simulink model "Test_Position_Joints"  (Simulink 6.5)
settings: Solver=FixedStepDiscrete  StartTime=0.0  StopTime=inf  FixedStep=0.025  RelTol=1e-3
libraries: xpclib x8, simulink x4
settings Model: Creator=ilMaggia  LastModifiedBy=ilMaggia
settings DebuggingCC: MultiTaskDSMMsg=warning  MultiTaskCondExecSysMsg=none
settings RTWCC: SystemTargetFile=rtwin.tlc  TemplateMakefile=rtwin.tmf  Description=Real-Time Windows Target  ProcessScript=rtwin_make_rtw_hook  IncludeERTFirstTime=on
settings RTWinTargetCC: TargetFcnLib=ansi_tfl_tmw.mat  GenFloatMathFcnCalls=ANSI_C  ModelReferenceCompliant=off  CCOptimize=on

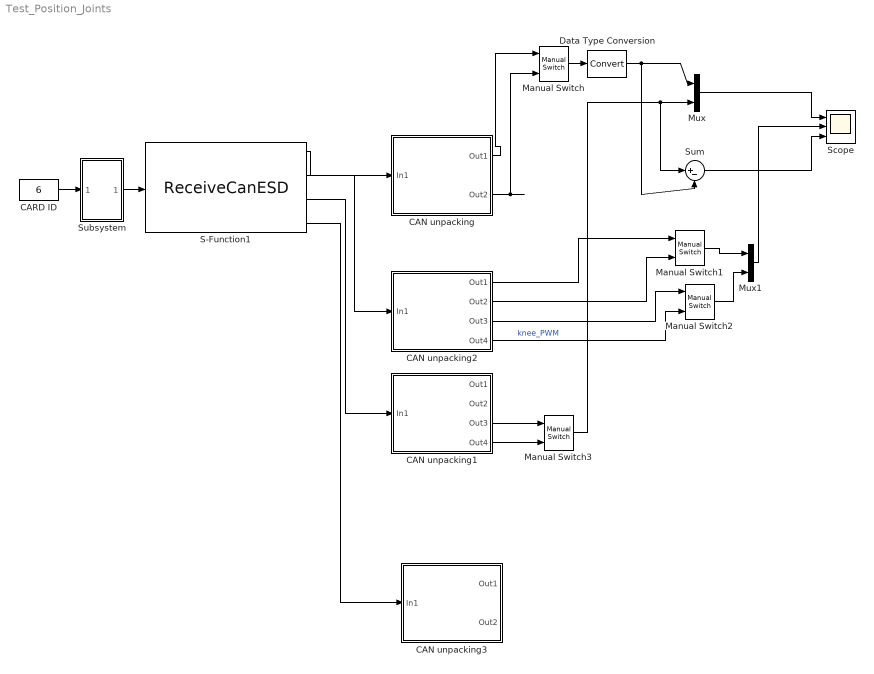
== system Test_Position_Joints ==
  CAN unpacking : Subsystem
  CAN unpacking1 : Subsystem
  CAN unpacking2 : Subsystem
  CAN unpacking3 : Subsystem
  CARD ID : Constant  Value=6  OutDataType=sfix(16)  ConRadixGroup=Use specified scaling  OutScaling=2^0  SampleTime=inf  FramePeriod=inf
  Data Type Conversion : DataTypeConversion
  Manual Switch{,1..3} (4 alike) : simulink/Signal Routing/Manual Switch  SystemSampleTime=-1  sw=1  action=0
  Mux : Mux  Inputs=2
  Mux1 : Mux  Inputs=2
  S-Function1 : S-Function  FunctionName=ReceiveCanESD  Parameters=0,0
  Scope : Scope  NumInputPorts=3
      settings: TimeRange=1000  YMin=0~-20~-50  YMax=2500~20~40  MaxDataPoints=50000
  Subsystem : Subsystem
  Sum : Sum  Inputs=|+-
  wires:
  CAN unpacking/1(Out1) -> Manual Switch/1
  CAN unpacking/2(Out2) -> Manual Switch/2
  S-Function1/1 -> CAN unpacking/1(In1)
  S-Function1/2 -> CAN unpacking2/1(In1)
  S-Function1/3 -> CAN unpacking1/1(In1)
  S-Function1/4 -> CAN unpacking3/1(In1)
  Mux/1 -> Scope/1
  Data Type Conversion/1 -> Mux/1, Sum/2
  Mux1/1 -> Scope/2
  Sum/1 -> Scope/3
  Manual Switch/1 -> Data Type Conversion/1
  Manual Switch1/1 -> Mux1/1
  CAN unpacking2/1(Out1) -> Manual Switch1/1
  Manual Switch2/1 -> Mux1/2
  CAN unpacking2/4(Out4) -> Manual Switch2/2  "knee_PWM"
  Manual Switch3/1 -> Mux/2, Sum/1
  CAN unpacking1/3(Out3) -> Manual Switch3/1
  CAN unpacking1/4(Out4) -> Manual Switch3/2
  Subsystem/1(Out1) -> S-Function1/1
  CARD ID/1 -> Subsystem/1(In1)
  CAN unpacking2/2(Out2) -> Manual Switch1/2
  CAN unpacking2/3(Out3) -> Manual Switch2/1

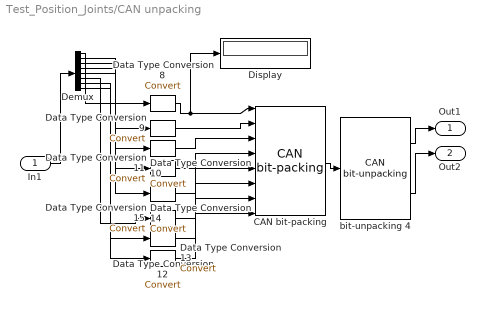
== system Test_Position_Joints/CAN unpacking ==
  In1 : Inport
  " bit-unpacking 4" : xpclib/CAN/Utilities/CAN bit-unpacking   bitpatterns={ [0:31] [32:63]}  dtypes={ 'int32' 'int32' }
  "CAN bit-packing " : xpclib/CAN/Utilities/CAN bit-packing   bitpatterns={ [0:7] [8:15] [16:23] [24:31] [32:39] [40:47] [48:55] [56:63] }
  Data Type Conversion{8..15} (8 alike) : DataTypeConversion  OutDataTypeMode=uint8
  Demux : Demux  Outputs=8
  Display : Display
  Out1 : Outport
  Out2 : Outport  Port=2
  wires:
  "CAN bit-packing "/1 -> " bit-unpacking 4"/1
  Data Type Conversion8/1 -> "CAN bit-packing "/1, Display/1
  Data Type Conversion9/1 -> "CAN bit-packing "/2
  Data Type Conversion10/1 -> "CAN bit-packing "/3
  Data Type Conversion11/1 -> "CAN bit-packing "/4
  Data Type Conversion14/1 -> "CAN bit-packing "/5
  Data Type Conversion15/1 -> "CAN bit-packing "/6
  Data Type Conversion12/1 -> "CAN bit-packing "/7
  Data Type Conversion13/1 -> "CAN bit-packing "/8
  Demux/1 -> Data Type Conversion8/1
  Demux/2 -> Data Type Conversion9/1
  Demux/3 -> Data Type Conversion10/1
  Demux/4 -> Data Type Conversion11/1
  Demux/5 -> Data Type Conversion14/1
  Demux/6 -> Data Type Conversion15/1
  Demux/7 -> Data Type Conversion12/1
  Demux/8 -> Data Type Conversion13/1
  " bit-unpacking 4"/1 -> Out1/1
  " bit-unpacking 4"/2 -> Out2/1
  In1/1 -> Demux/1

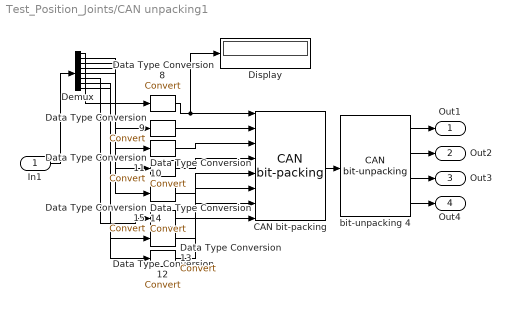
== system Test_Position_Joints/CAN unpacking1 ==
  In1 : Inport
  " bit-unpacking 4" : xpclib/CAN/Utilities/CAN bit-unpacking   bitpatterns={ [0:15] [16:31] [32:47] [48:63]}  dtypes={ 'int16' 'int16' 'int16' 'int16'}
  "CAN bit-packing " : xpclib/CAN/Utilities/CAN bit-packing   bitpatterns={ [0:7] [8:15] [16:23] [24:31] [32:39] [40:47] [48:55] [56:63] }
  Data Type Conversion{8..15} (8 alike) : DataTypeConversion  OutDataTypeMode=uint8
  Demux : Demux  Outputs=8
  Display : Display
  Out1 : Outport
  Out2 : Outport  Port=2
  Out3 : Outport  Port=3
  Out4 : Outport  Port=4
  wires:
  " bit-unpacking 4"/4 -> Out4/1
  " bit-unpacking 4"/3 -> Out3/1
  In1/1 -> Demux/1
  " bit-unpacking 4"/2 -> Out2/1
  " bit-unpacking 4"/1 -> Out1/1
  Demux/8 -> Data Type Conversion13/1
  Demux/7 -> Data Type Conversion12/1
  Demux/6 -> Data Type Conversion15/1
  Demux/5 -> Data Type Conversion14/1
  Demux/4 -> Data Type Conversion11/1
  Demux/3 -> Data Type Conversion10/1
  Demux/2 -> Data Type Conversion9/1
  Demux/1 -> Data Type Conversion8/1
  Data Type Conversion13/1 -> "CAN bit-packing "/8
  Data Type Conversion12/1 -> "CAN bit-packing "/7
  Data Type Conversion15/1 -> "CAN bit-packing "/6
  Data Type Conversion14/1 -> "CAN bit-packing "/5
  Data Type Conversion11/1 -> "CAN bit-packing "/4
  Data Type Conversion10/1 -> "CAN bit-packing "/3
  Data Type Conversion9/1 -> "CAN bit-packing "/2
  Data Type Conversion8/1 -> Display/1, "CAN bit-packing "/1
  "CAN bit-packing "/1 -> " bit-unpacking 4"/1

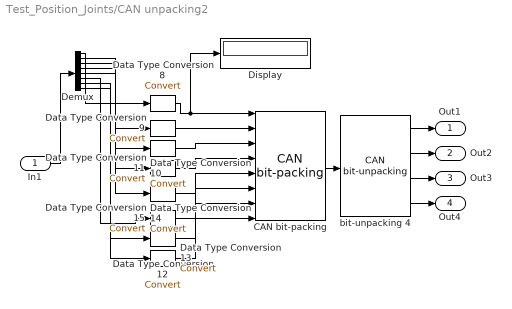
== system Test_Position_Joints/CAN unpacking2 ==
  In1 : Inport
  " bit-unpacking 4" : xpclib/CAN/Utilities/CAN bit-unpacking   bitpatterns={ [0:15] [16:31] [32:47] [48:63]}  dtypes={ 'int16' 'int16' 'int16' 'int16'}
  "CAN bit-packing " : xpclib/CAN/Utilities/CAN bit-packing   bitpatterns={ [0:7] [8:15] [16:23] [24:31] [32:39] [40:47] [48:55] [56:63] }
  Data Type Conversion{8..15} (8 alike) : DataTypeConversion  OutDataTypeMode=uint8
  Demux : Demux  Outputs=8
  Display : Display
  Out1 : Outport
  Out2 : Outport  Port=2
  Out3 : Outport  Port=3
  Out4 : Outport  Port=4
  wires:
  "CAN bit-packing "/1 -> " bit-unpacking 4"/1
  Data Type Conversion8/1 -> "CAN bit-packing "/1, Display/1
  Data Type Conversion9/1 -> "CAN bit-packing "/2
  Data Type Conversion10/1 -> "CAN bit-packing "/3
  Data Type Conversion11/1 -> "CAN bit-packing "/4
  Data Type Conversion14/1 -> "CAN bit-packing "/5
  Data Type Conversion15/1 -> "CAN bit-packing "/6
  Data Type Conversion12/1 -> "CAN bit-packing "/7
  Data Type Conversion13/1 -> "CAN bit-packing "/8
  Demux/1 -> Data Type Conversion8/1
  Demux/2 -> Data Type Conversion9/1
  Demux/3 -> Data Type Conversion10/1
  Demux/4 -> Data Type Conversion11/1
  Demux/5 -> Data Type Conversion14/1
  Demux/6 -> Data Type Conversion15/1
  Demux/7 -> Data Type Conversion12/1
  Demux/8 -> Data Type Conversion13/1
  " bit-unpacking 4"/1 -> Out1/1
  " bit-unpacking 4"/2 -> Out2/1
  In1/1 -> Demux/1
  " bit-unpacking 4"/3 -> Out3/1
  " bit-unpacking 4"/4 -> Out4/1

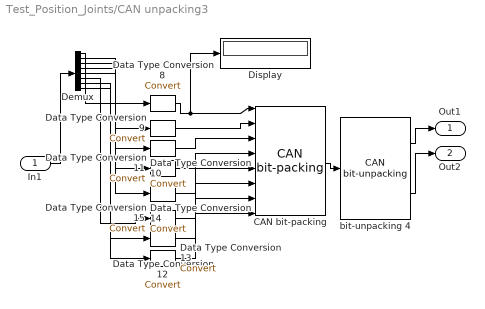
== system Test_Position_Joints/CAN unpacking3 ==
  In1 : Inport
  " bit-unpacking 4" : xpclib/CAN/Utilities/CAN bit-unpacking   bitpatterns={ [0:31] [32:63]}  dtypes={ 'int32' 'int32' }
  "CAN bit-packing " : xpclib/CAN/Utilities/CAN bit-packing   bitpatterns={ [0:7] [8:15] [16:23] [24:31] [32:39] [40:47] [48:55] [56:63] }
  Data Type Conversion{8..15} (8 alike) : DataTypeConversion  OutDataTypeMode=uint8
  Demux : Demux  Outputs=8
  Display : Display
  Out1 : Outport
  Out2 : Outport  Port=2
  wires:
  "CAN bit-packing "/1 -> " bit-unpacking 4"/1
  Data Type Conversion8/1 -> "CAN bit-packing "/1, Display/1
  Data Type Conversion9/1 -> "CAN bit-packing "/2
  Data Type Conversion10/1 -> "CAN bit-packing "/3
  Data Type Conversion11/1 -> "CAN bit-packing "/4
  Data Type Conversion14/1 -> "CAN bit-packing "/5
  Data Type Conversion15/1 -> "CAN bit-packing "/6
  Data Type Conversion12/1 -> "CAN bit-packing "/7
  Data Type Conversion13/1 -> "CAN bit-packing "/8
  Demux/1 -> Data Type Conversion8/1
  Demux/2 -> Data Type Conversion9/1
  Demux/3 -> Data Type Conversion10/1
  Demux/4 -> Data Type Conversion11/1
  Demux/5 -> Data Type Conversion14/1
  Demux/6 -> Data Type Conversion15/1
  Demux/7 -> Data Type Conversion12/1
  Demux/8 -> Data Type Conversion13/1
  " bit-unpacking 4"/1 -> Out1/1
  " bit-unpacking 4"/2 -> Out2/1
  In1/1 -> Demux/1

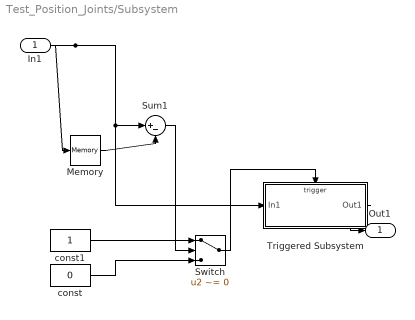
== system Test_Position_Joints/Subsystem ==
  In1 : Inport
  Memory : Memory
  Sum1 : Sum  Inputs=|+-
  Switch : Switch  Criteria=u2 ~= 0
  Triggered Subsystem : Subsystem  TreatAsAtomicUnit=on
  const : Constant  Value=0  OutDataType=sfix(16)  ConRadixGroup=Use specified scaling  OutScaling=2^0  SampleTime=inf  FramePeriod=inf
  const1 : Constant  Value=1  OutDataType=sfix(16)  ConRadixGroup=Use specified scaling  OutScaling=2^0  SampleTime=inf  FramePeriod=inf
  Out1 : Outport
  wires:
  Switch/1 -> Triggered Subsystem/Trigger
  In1/1 -> Triggered Subsystem/1(In1), Sum1/1, Memory/1
  const1/1 -> Switch/1
  const/1 -> Switch/3
  Memory/1 -> Sum1/2
  Sum1/1 -> Switch/2
  Triggered Subsystem/1(Out1) -> Out1/1

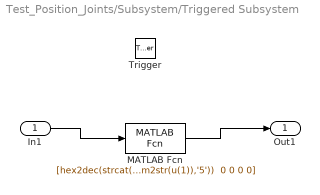
== system Test_Position_Joints/Subsystem/Triggered Subsystem ==
  In1 : Inport
  Trigger : TriggerPort
  MATLAB Fcn : MATLABFcn  MATLABFcn="[hex2dec(strcat('1',num2str(u(1)),'1'))  hex2dec(strcat('1',num2str(u(1)),'2')) hex2dec(strcat('1',num2str(u(1)),'4') ) hex2dec(strcat('1',num2str(u(1)),'5'))  0 0 0 0]"
  Out1 : Outport
  wires:
  In1/1 -> MATLAB Fcn/1
  MATLAB Fcn/1 -> Out1/1
